simulink model "Boot_loagic"  (R2020a)
settings: Solver=FixedStepDiscrete  StartTime=0.0  StopTime=50  FixedStep=1  RelTol=1e-3
settings Model: Creator=sgrak  LastModifiedBy=sgrak

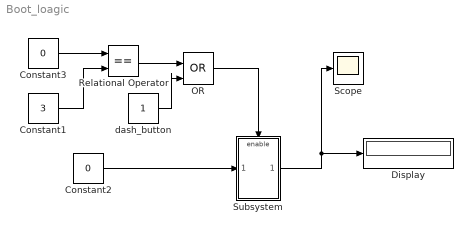
== system Boot_loagic ==
  Constant1 : Constant  Value=3
  Constant2 : Constant  Value=0
  Constant3 : Constant  Value=0
  Display : Display
  OR : Logic  Operator=OR  IconShape=distinctive  AllPortsSameDT=off  OutDataTypeStr=boolean
  Relational Operator : RelationalOperator  Operator===  OutDataTypeStr=boolean  RndMeth=Simplest
  Scope : Scope
  Subsystem : Subsystem
  dash_button : Constant
  wires:
  Constant2/1 -> Subsystem/1(In1)
  Constant1/1 -> Relational Operator/2
  Subsystem/1(Output) -> Scope/1, Display/1
  Relational Operator/1 -> OR/1
  dash_button/1 -> OR/2
  OR/1 -> Subsystem/Enable
  Constant3/1 -> Relational Operator/1

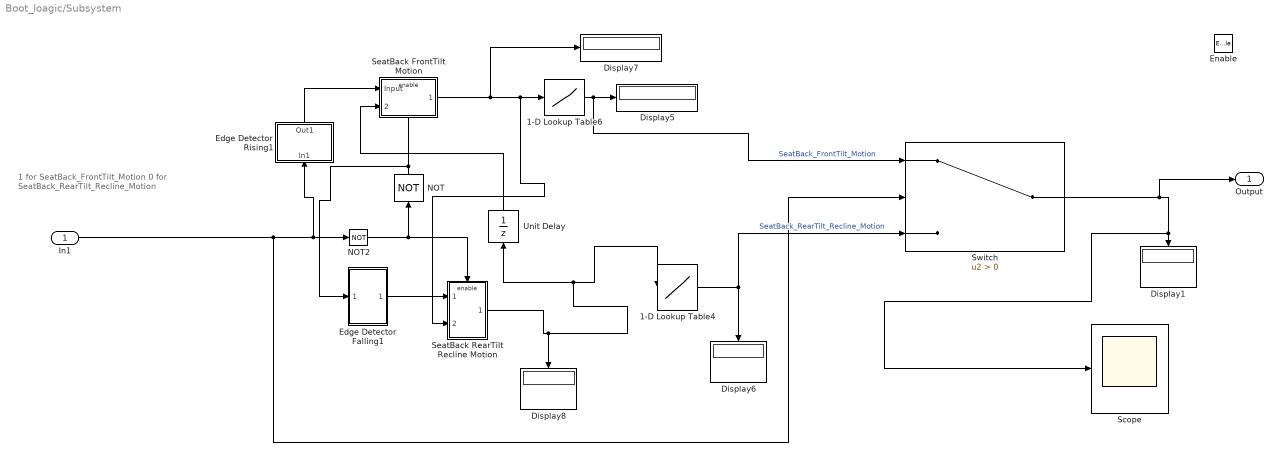
== system Boot_loagic/Subsystem ==
  note: 1 for SeatBack_FrontTilt_Motion
      | 0 for SeatBack_RearTilt_Recline_Motion
  In1 : Inport
  Enable : EnablePort
  1-D Lookup Table4 : Lookup_n-D  NumberOfTableDimensions=1  BreakpointsForDimension1=[500 1000 1600]  Table=[0 45 90]  InternalRulePriority=Speed  RndMeth=Simplest  InputSameDT=on
  1-D Lookup Table6 : Lookup_n-D  NumberOfTableDimensions=1  BreakpointsForDimension1=[500 1000 1600]  Table=[0 45 90]  InternalRulePriority=Speed  RndMeth=Simplest  InputSameDT=on
  Display{1,5..8} (5 alike) : Display
  Edge Detector Falling1 : Subsystem  TreatAsAtomicUnit=on
  Edge Detector Rising1 : Subsystem  TreatAsAtomicUnit=on
  NOT : Logic  Operator=NOT  IconShape=distinctive  AllPortsSameDT=off  OutDataTypeStr=boolean
  NOT2 : Logic  Operator=NOT  IconShape=distinctive  AllPortsSameDT=off  OutDataTypeStr=boolean
  Scope : Scope
  SeatBack FrontTilt Motion : Subsystem
  SeatBack RearTilt Recline Motion : Subsystem
  Switch : Switch  Criteria=u2 > Threshold
  Unit Delay : UnitDelay  SampleTime=-1  HasFrameUpgradeWarning=on
  Output : Outport
  wires:
  SeatBack FrontTilt Motion/1(Output1) -> Display7/1, 1-D Lookup Table6/1, SeatBack RearTilt Recline Motion/2(Input1)
  In1/1 -> Switch/2, Edge Detector Rising1/1(In1), NOT2/1
  NOT2/1 -> SeatBack RearTilt Recline Motion/Enable, NOT/1
  Switch/1 -> Output/1, Display1/1, Scope/1
  1-D Lookup Table4/1 -> Switch/3, Display6/1  "SeatBack_RearTilt_Recline_Motion"
  Edge Detector Rising1/1(Out1) -> SeatBack FrontTilt Motion/1(Input)
  SeatBack RearTilt Recline Motion/1(Output) -> 1-D Lookup Table4/1, Unit Delay/1, Display8/1
  Unit Delay/1 -> SeatBack FrontTilt Motion/2(Input1)
  Edge Detector Falling1/1(Input) -> SeatBack RearTilt Recline Motion/1(Input)
  1-D Lookup Table6/1 -> Switch/1, Display5/1  "SeatBack_FrontTilt_Motion"
  NOT/1 -> Edge Detector Falling1/1(In1), SeatBack FrontTilt Motion/Enable

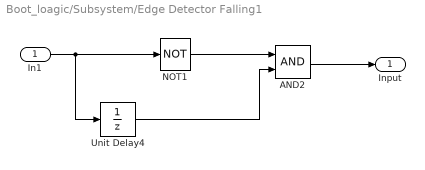
== system Boot_loagic/Subsystem/Edge Detector Falling1 ==
  In1 : Inport
  AND2 : Logic  AllPortsSameDT=off  OutDataTypeStr=boolean
  NOT1 : Logic  Operator=NOT  IconShape=distinctive  AllPortsSameDT=off  OutDataTypeStr=boolean
  Unit Delay4 : UnitDelay  InitialCondition=1  SampleTime=-1  HasFrameUpgradeWarning=on
  Input : Outport
  wires:
  AND2/1 -> Input/1
  In1/1 -> NOT1/1, Unit Delay4/1
  Unit Delay4/1 -> AND2/2
  NOT1/1 -> AND2/1

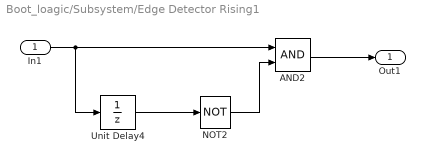
== system Boot_loagic/Subsystem/Edge Detector Rising1 ==
  In1 : Inport
  AND2 : Logic  AllPortsSameDT=off  OutDataTypeStr=boolean
  NOT2 : Logic  Operator=NOT  IconShape=distinctive  AllPortsSameDT=off  OutDataTypeStr=boolean
  Unit Delay4 : UnitDelay  InitialCondition=1  SampleTime=-1  HasFrameUpgradeWarning=on
  Out1 : Outport
  wires:
  NOT2/1 -> AND2/2
  In1/1 -> Unit Delay4/1, AND2/1
  Unit Delay4/1 -> NOT2/1
  AND2/1 -> Out1/1

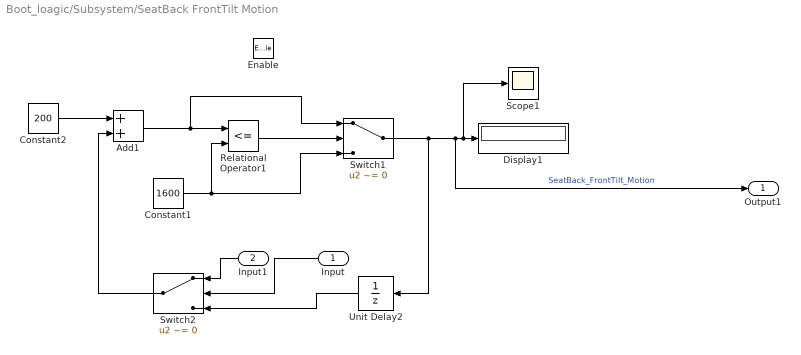
== system Boot_loagic/Subsystem/SeatBack FrontTilt Motion ==
  Input : Inport
  Input1 : Inport  Port=2
  Enable : EnablePort
  Add1 : Sum
  Constant1 : Constant  Value=1600
  Constant2 : Constant  Value=200
  Display1 : Display
  Relational Operator1 : RelationalOperator  Operator=<=  OutDataTypeStr=boolean  RndMeth=Simplest
  Scope1 : Scope
  Switch1 : Switch  Criteria=u2 ~= 0
  Switch2 : Switch  Criteria=u2 ~= 0
  Unit Delay2 : UnitDelay  InitialCondition=300  SampleTime=-1  HasFrameUpgradeWarning=on
  Output1 : Outport
  wires:
  Constant1/1 -> Switch1/3, Relational Operator1/2
  Relational Operator1/1 -> Switch1/2
  Constant2/1 -> Add1/1
  Add1/1 -> Switch1/1, Relational Operator1/1
  Switch1/1 -> Unit Delay2/1, Output1/1, Scope1/1, Display1/1  "SeatBack_FrontTilt_Motion"
  Input1/1 -> Switch2/1
  Input/1 -> Switch2/2
  Unit Delay2/1 -> Switch2/3
  Switch2/1 -> Add1/2

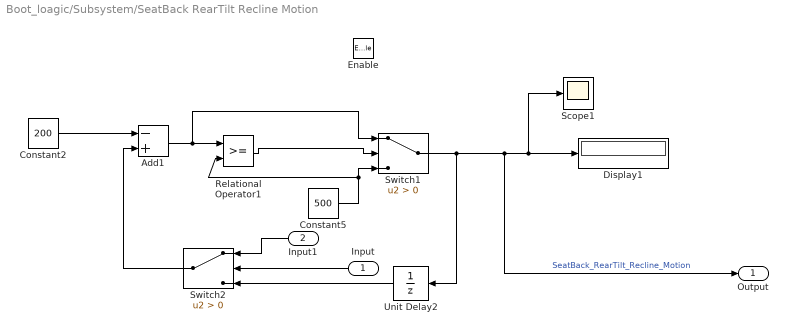
== system Boot_loagic/Subsystem/SeatBack RearTilt Recline Motion ==
  Input : Inport
  Input1 : Inport  Port=2
  Enable : EnablePort
  Add1 : Sum  Inputs=-+
  Constant2 : Constant  Value=200
  Constant5 : Constant  Value=500
  Display1 : Display
  Relational Operator1 : RelationalOperator  OutDataTypeStr=boolean  RndMeth=Simplest
  Scope1 : Scope
  Switch1 : Switch  Criteria=u2 > Threshold
  Switch2 : Switch  Criteria=u2 > Threshold
  Unit Delay2 : UnitDelay  InitialCondition=1500  SampleTime=-1  HasFrameUpgradeWarning=on
  Output : Outport
  wires:
  Relational Operator1/1 -> Switch1/2
  Constant2/1 -> Add1/1
  Add1/1 -> Switch1/1, Relational Operator1/1
  Constant5/1 -> Relational Operator1/2, Switch1/3
  Switch1/1 -> Unit Delay2/1, Output/1, Display1/1, Scope1/1  "SeatBack_RearTilt_Recline_Motion"
  Switch2/1 -> Add1/2
  Input1/1 -> Switch2/1
  Unit Delay2/1 -> Switch2/3
  Input/1 -> Switch2/2
